simulink model "MS02_SimModel_01"  (R2016b)
settings: Solver=ode1  StartTime=0.0  StopTime=10  RelTol=1e-3
values from neighbouring files (symbols this model uses):
  A = 40    [MS02_UAV_motion_turbulence_terrain.m]    (also in MS03_Statistical_analysis_trajectories.m = [ 0, -g*cos(mx(2,1)), 0, 0;          g/mx(1,1)^2*cos(mx(2,1))
  a1 = 23341 + i    [MS02_UAV_motion_turbulence_terrain.m]
  a2 = 24341 + i    [MS02_UAV_motion_turbulence_terrain.m]
  a3 = 25341 + i    [MS02_UAV_motion_turbulence_terrain.m]
  Erel = 5    [MS02_UAV_motion_turbulence_terrain.m]
  h0 = 60    [MS02_UAV_motion_turbulence_terrain.m]
  htr = 25    [MS02_UAV_motion_turbulence_terrain.m]
  K = 0.2    [MS02_UAV_motion_turbulence_terrain.m]
  Kd = 4.4552    [MS02_UAV_motion_turbulence_terrain.m]
  Ki = -0.0024    [MS02_UAV_motion_turbulence_terrain.m]
  Kp = 3.159    [MS02_UAV_motion_turbulence_terrain.m]
  Krel = 300    [MS02_UAV_motion_turbulence_terrain.m]
  l = L/V    (= 1.42857142857)    [MS02_UAV_motion_turbulence_terrain.m]
  Ot = 12    [MS02_UAV_motion_turbulence_terrain.m]
  T = 0.15    [MS02_UAV_motion_turbulence_terrain.m]
  Trel = 10    [MS02_UAV_motion_turbulence_terrain.m]
  V = 280    [MS02_UAV_motion_turbulence_terrain.m]
libraries: simulink x3
settings Model: Creator=Maksim  LastModifiedBy=Maksim

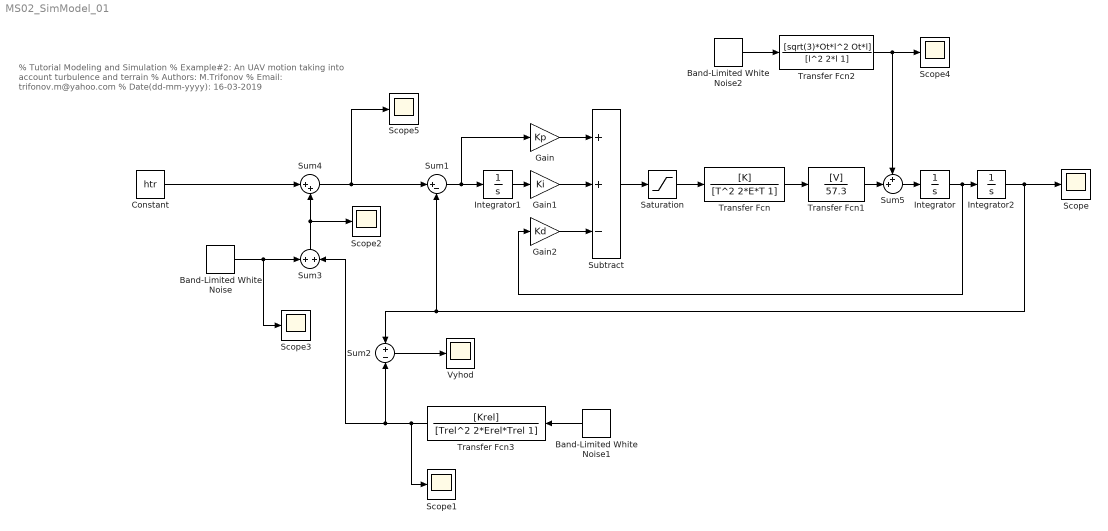
== system MS02_SimModel_01 ==
  note: % Tutorial Modeling and Simulation
      | % Example#2: An UAV motion taking into account turbulence and terrain
      | % Authors: M.Trifonov
      | % Email: trifonov.m@yahoo.com
      | % Date(dd-mm-yyyy): 16-03-2019
  Band-Limited White Noise : simulink/Sources/Band-Limited White Noise  Cov=[0.1]  Ts=0.1  seed=[a2]
  Band-Limited White Noise1 : simulink/Sources/Band-Limited White Noise  Cov=[0.1]  Ts=0.1  seed=[a3]
  Band-Limited White Noise2 : simulink/Sources/Band-Limited White Noise  Cov=[1]  Ts=0.1  seed=[a1]
  Constant : Constant  Value=htr
  Gain : Gain  Gain=Kp
  Gain1 : Gain  Gain=Ki
  Gain2 : Gain  Gain=Kd
  Integrator : Integrator
  Integrator1 : Integrator
  Integrator2 : Integrator  InitialCondition=h0
  Saturation : Saturate  UpperLimit=A  LowerLimit=-A
  Scope{,1..5} (6 alike) : Scope
  Subtract : Sum  Inputs=++-
  Sum1 : Sum  Inputs=|+-
  Sum2 : Sum  Inputs=+|-
  Sum3 : Sum  Inputs=+|+
  Sum4 : Sum  Inputs=|++
  Sum5 : Sum  Inputs=++|
  Transfer Fcn : TransferFcn  Numerator=[K]  Denominator=[T^2 2*E*T 1]
  Transfer Fcn1 : TransferFcn  Numerator=[V]  Denominator=[57.3]
  Transfer Fcn2 : TransferFcn  Numerator=[sqrt(3)*Ot*l^2 Ot*l]  Denominator=[l^2 2*l 1]
  Transfer Fcn3 : TransferFcn  Numerator=[Krel]  Denominator=[Trel^2 2*Erel*Trel 1]
  Vyhod : Scope
  wires:
  Gain/1 -> Subtract/1
  Gain1/1 -> Subtract/2
  Integrator1/1 -> Gain1/1
  Sum1/1 -> Gain/1, Integrator1/1
  Integrator2/1 -> Sum2/1, Sum1/2, Scope/1
  Integrator/1 -> Gain2/1, Integrator2/1
  Subtract/1 -> Saturation/1
  Transfer Fcn/1 -> Transfer Fcn1/1
  Transfer Fcn3/1 -> Scope1/1, Sum2/2, Sum3/2
  Constant/1 -> Sum4/1
  Sum3/1 -> Scope2/1, Sum4/2
  Sum4/1 -> Scope5/1, Sum1/1
  Band-Limited White Noise/1 -> Sum3/1, Scope3/1
  Band-Limited White Noise1/1 -> Transfer Fcn3/1
  Sum2/1 -> Vyhod/1
  Transfer Fcn1/1 -> Sum5/2
  Sum5/1 -> Integrator/1
  Band-Limited White Noise2/1 -> Transfer Fcn2/1
  Transfer Fcn2/1 -> Scope4/1, Sum5/1
  Gain2/1 -> Subtract/3
  Saturation/1 -> Transfer Fcn/1
